simulink model "roombaSensorsExample"  (R2017b)
settings: Solver=VariableStepAuto  StartTime=0.0  StopTime=10.0  RelTol=1e-3
libraries: roombaCtrl x1
settings Model: Creator=wafflefries  LastModifiedBy=wafflefries

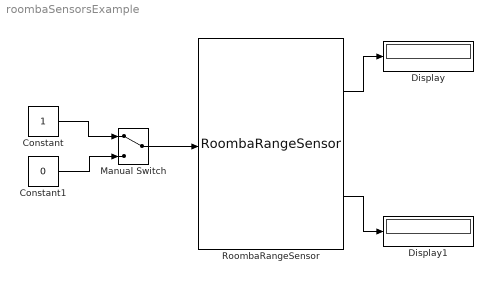
== system roombaSensorsExample ==
  Constant : Constant
  Constant1 : Constant  Value=0
  Display : Display
  Display1 : Display
  Manual Switch : ManualSwitch
  RoombaRangeSensor : roombaCtrl/RoombaRangeSensor
  wires:
  Manual Switch/1 -> RoombaRangeSensor/1
  Constant/1 -> Manual Switch/1
  Constant1/1 -> Manual Switch/2
  RoombaRangeSensor/1 -> Display/1
  RoombaRangeSensor/2 -> Display1/1
